simulink model "HT07_accumulator_thermal_model"  (R2022a)
settings: Solver=VariableStepAuto  StartTime=0.0  StopTime=Tend  RelTol=1e-7  AbsTol=1e-7
values from neighbouring files (symbols this model uses):
  AH = 14    [HT07_Simulink_Setup.m]
  SOC0 = 1    [HT07_Simulink_Setup.m]
  startTempC = 25    [HT07_Simulink_Setup.m]
  tabResis = 0.00009    (= 9e-05)    [HT07_Simulink_Setup.m]
undefined symbols (not defined in the file or in its folder): DiscIntNeverNeededParam
libraries: fl_lib x50, nesl_utility x16, ee_lib x2
settings Model: Creator=elrii  LastModifiedBy=David
settings SolverCC: AutoScaleAbsTol=off  AlgebraicLoopSolver=TrustRegion
settings DataIOCC: ReturnWorkspaceOutputsName=tp141c3138_a421_409b_bff7_0e00beb78378
settings DebuggingCC: UnconnectedInputMsg=warning  UnconnectedOutputMsg=warning  UnconnectedLineMsg=warning  SymbolicDimsDataTypeCodeGenerationDiagnostic=none  SFMachineParentedDataDiag=warning
settings SFSimCC: CustomCodeUndefinedFunction=UseInterfaceOnly
settings RTWCC: DLArmComputeVersion=19.05
settings SimscapeCC: SimscapeLogType=all  SimscapeLogSimulationStatistics=on  SimscapeLogDataHistory=10000

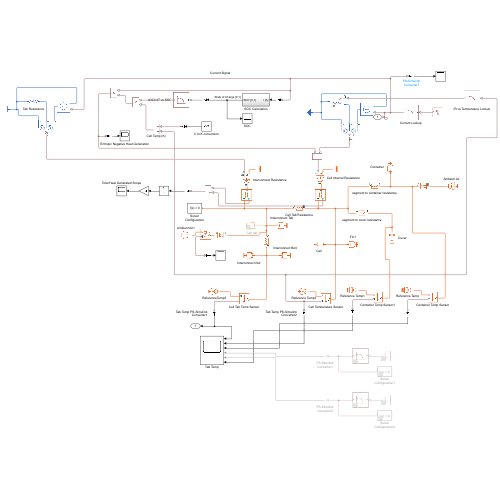
[thumbnail: Simulink's stored preview of the top-level diagram]
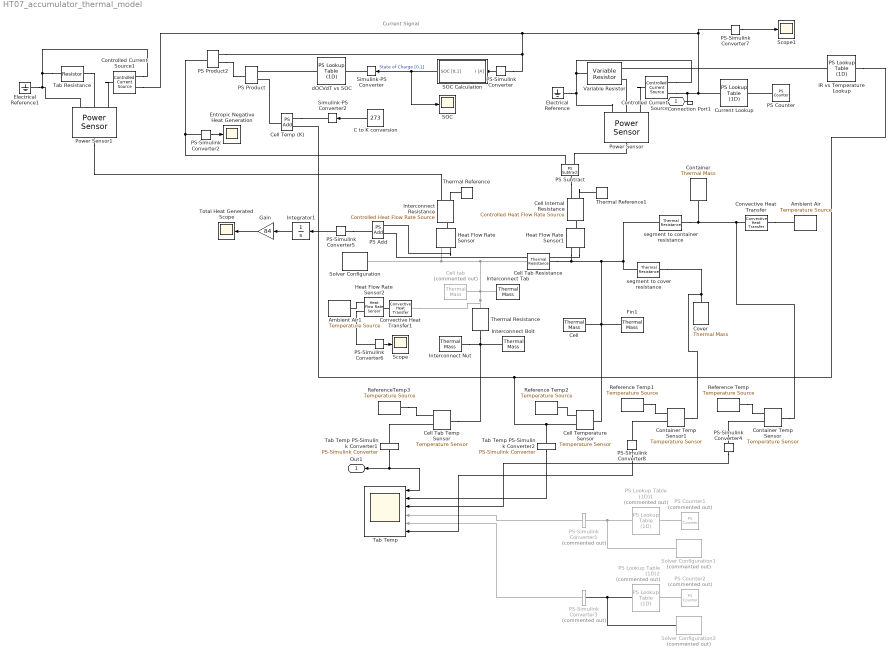
== system HT07_accumulator_thermal_model ==
  note: Current Signal
  " Fin1" : fl_lib/Thermal/Thermal Elements/Thermal Mass  mass=mFin kg  sp_heat=cAl J/kg/K  T_specify=on  T_priority=High  T=startTempC degC  T_nominal_specify=off  T_nominal_unit=K  T_nominal_value=1  Q_specify=off  Q_priority=None  Q=0 W  Q_nominal_specify=off  Q_nominal_unit=W  Q_nominal_value=1
      settings: SourceProductBaseCode=PW,SS,VE
  Ambient Air : fl_lib/Thermal/Thermal Sources/Temperature Source  temperature=startTempC degC
      settings: SourceProductBaseCode=PW,SS,VE
  Ambient Air1 : fl_lib/Thermal/Thermal Sources/Temperature Source  temperature=startTempC degC
      settings: SourceProductBaseCode=PW,SS,VE
  C to K conversion : Constant  Value=273
  "Cell " : fl_lib/Thermal/Thermal Elements/Thermal Mass  mass=mCell kg  sp_heat=cCell J/kg/K  T_specify=on  T_priority=High  T=startTempC degC  T_nominal_specify=off  T_nominal_unit=K  T_nominal_value=1  Q_specify=off  Q_priority=None  Q=0 W  Q_nominal_specify=off  Q_nominal_unit=W  Q_nominal_value=1
      settings: SourceProductBaseCode=PW,SS,VE
  Cell Internal Resistance : fl_lib/Thermal/Thermal Sources/Controlled Heat Flow Rate Source
      settings: SourceProductBaseCode=PW,SS,VE
  Cell Tab Resistance : fl_lib/Thermal/Thermal Elements/Thermal Resistance  resistance=R_tc K/W  T_specify=off  T_priority=None  T=0 K  T_nominal_specify=off  T_nominal_unit=K  T_nominal_value=1  Q_specify=off  Q_priority=None  Q=0 W  Q_nominal_specify=off  Q_nominal_unit=W  Q_nominal_value=1
      settings: SourceProductBaseCode=PW,SS,VE
  Cell Tab Temp Sensor : fl_lib/Thermal/Thermal Sensors/Temperature Sensor
      settings: SourceProductBaseCode=PW,SS,VE
  Cell Temp (K) : fl_lib/Physical Signals/Functions/PS Add
      settings: SourceProductBaseCode=PW,SS,VE
  Cell Temperature Sensor : fl_lib/Thermal/Thermal Sensors/Temperature Sensor
      settings: SourceProductBaseCode=PW,SS,VE
  Cell tab : fl_lib/Thermal/Thermal Elements/Thermal Mass  Commented=on  mass=cellTabThermalMass kg  sp_heat=cCu J/kg/K  T_specify=on  T_priority=High  T=startTempC degC  T_nominal_specify=off  T_nominal_unit=K  T_nominal_value=1  Q_specify=off  Q_priority=None  Q=0 W  Q_nominal_specify=off  Q_nominal_unit=W  Q_nominal_value=1
      settings: SourceProductBaseCode=PW,SS,VE
  Container : fl_lib/Thermal/Thermal Elements/Thermal Mass  mass=mContainerAdj kg  sp_heat=cAl J/kg/K  T_specify=on  T_priority=High  T=startTempC degC  T_nominal_specify=off  T_nominal_unit=K  T_nominal_value=1  Q_specify=off  Q_priority=None  Q=0 W  Q_nominal_specify=off  Q_nominal_unit=W  Q_nominal_value=1
      settings: SourceProductBaseCode=PW,SS,VE
  Container Temp Sensor : fl_lib/Thermal/Thermal Sensors/Temperature Sensor
      settings: SourceProductBaseCode=PW,SS,VE
  Container Temp Sensor1 : fl_lib/Thermal/Thermal Sensors/Temperature Sensor
      settings: SourceProductBaseCode=PW,SS,VE
  Controlled Current Source : fl_lib/Electrical/Electrical Sources/Controlled Current Source
      settings: SourceProductBaseCode=PW,SS,VE
  Controlled Current Source1 : fl_lib/Electrical/Electrical Sources/Controlled Current Source
      settings: SourceProductBaseCode=PW,SS,VE
  Convective Heat Transfer : fl_lib/Thermal/Thermal Elements/Convective Heat Transfer  area=convectionArea m^2  heat_tr_coeff=20 W/(m^2*K)  T_specify=off  T_priority=None  T=0 K  T_nominal_specify=off  T_nominal_unit=K  T_nominal_value=1  Q_specify=off  Q_priority=None  Q=0 W  Q_nominal_specify=off  Q_nominal_unit=W  Q_nominal_value=1
      settings: SourceProductBaseCode=PW,SS,VE
  Convective Heat Transfer1 : fl_lib/Thermal/Thermal Elements/Convective Heat Transfer  area=tabConvectionArea m^2  heat_tr_coeff=100 W/(m^2*K)  T_specify=off  T_priority=None  T=0 K  T_nominal_specify=off  T_nominal_unit=K  T_nominal_value=1  Q_specify=off  Q_priority=None  Q=0 W  Q_nominal_specify=off  Q_nominal_unit=W  Q_nominal_value=1
      settings: SourceProductBaseCode=PW,SS,VE
  Cover : fl_lib/Thermal/Thermal Elements/Thermal Mass  mass=mCoverAdj kg  sp_heat=cAl J/kg/K  T_specify=on  T_priority=High  T=startTempC degC  T_nominal_specify=off  T_nominal_unit=K  T_nominal_value=1  Q_specify=off  Q_priority=None  Q=0 W  Q_nominal_specify=off  Q_nominal_unit=W  Q_nominal_value=1
      settings: SourceProductBaseCode=PW,SS,VE
  Current Lookup : fl_lib/Physical Signals/Lookup Tables/PS Lookup Table (1D)  x=time  f=current A  interp_method=simscape.enum.interpolation.linear  extrap_method=simscape.enum.extrapolation.nearest
      settings: SourceProductBaseCode=PW,SS,VE
  Electrical Reference : fl_lib/Electrical/Electrical Elements/Electrical Reference
      settings: SourceProductBaseCode=PW,SS,VE
  Electrical Reference1 : fl_lib/Electrical/Electrical Elements/Electrical Reference
      settings: SourceProductBaseCode=PW,SS,VE
  Entropic Negative Heat Generation : Scope
  Gain : Gain  Gain=84
  Heat Flow Rate Sensor : fl_lib/Thermal/Thermal Sensors/Heat Flow Rate Sensor
      settings: SourceProductBaseCode=PW,SS,VE
  Heat Flow Rate Sensor1 : fl_lib/Thermal/Thermal Sensors/Heat Flow Rate Sensor
      settings: SourceProductBaseCode=PW,SS,VE
  Heat Flow Rate Sensor2 : fl_lib/Thermal/Thermal Sensors/Heat Flow Rate Sensor
      settings: SourceProductBaseCode=PW,SS,VE
  IR vs Temperature Lookup : fl_lib/Physical Signals/Lookup Tables/PS Lookup Table (1D)  x=tempVec K  f=IRVec Ohm  interp_method=simscape.enum.interpolation.linear  extrap_method=simscape.enum.extrapolation.nearest
      settings: SourceProductBaseCode=PW,SS,VE
  Integrator1 : Integrator
  Interconnect Bolt : fl_lib/Thermal/Thermal Elements/Thermal Mass  mass=mInterconnectBoltTotal kg  sp_heat=cSt J/kg/K  T_specify=on  T_priority=High  T=startTempC degC  T_nominal_specify=off  T_nominal_unit=K  T_nominal_value=1  Q_specify=off  Q_priority=None  Q=0 W  Q_nominal_specify=off  Q_nominal_unit=W  Q_nominal_value=1
      settings: SourceProductBaseCode=PW,SS,VE
  Interconnect Nut : fl_lib/Thermal/Thermal Elements/Thermal Mass  mass=mInterconnectNutTotal kg  sp_heat=cSt J/kg/K  T_specify=on  T_priority=High  T=startTempC degC  T_nominal_specify=off  T_nominal_unit=K  T_nominal_value=1  Q_specify=off  Q_priority=None  Q=0 W  Q_nominal_specify=off  Q_nominal_unit=W  Q_nominal_value=1
      settings: SourceProductBaseCode=PW,SS,VE
  Interconnect Resistance : fl_lib/Thermal/Thermal Sources/Controlled Heat Flow Rate Source
      settings: SourceProductBaseCode=PW,SS,VE
  Interconnect Tab : fl_lib/Thermal/Thermal Elements/Thermal Mass  mass=mInterconnect kg  sp_heat=cAl J/kg/K  T_specify=on  T_priority=High  T=startTempC degC  T_nominal_specify=off  T_nominal_unit=K  T_nominal_value=1  Q_specify=off  Q_priority=None  Q=0 W  Q_nominal_specify=off  Q_nominal_unit=W  Q_nominal_value=1
      settings: SourceProductBaseCode=PW,SS,VE
  PS Add : fl_lib/Physical Signals/Functions/PS Add
      settings: SourceProductBaseCode=PW,SS,VE
  PS Counter : fl_lib/Physical Signals/Sources/PS Counter  sample_time=1 s  init_val=1  reset_val=0  max_val=100000
      settings: SourceProductBaseCode=PW,SS,VE  InternalSimscapePortConfiguration="{\"Bottom\":[],\"Left\":[],\"Right\":[{\"id\":\"Y\",\"label\":\"Y\",\"type\":\"output\"}],\"Top\":[]}"
  PS Counter1 : fl_lib/Physical Signals/Sources/PS Counter  Commented=on  sample_time=1 s  init_val=1  reset_val=0  max_val=100000
      settings: SourceProductBaseCode=PW,SS,VE  InternalSimscapePortConfiguration="{\"Bottom\":[],\"Left\":[],\"Right\":[{\"id\":\"Y\",\"label\":\"Y\",\"type\":\"output\"}],\"Top\":[]}"
  PS Counter2 : fl_lib/Physical Signals/Sources/PS Counter  Commented=on  sample_time=1 s  init_val=1  reset_val=0  max_val=100000
      settings: SourceProductBaseCode=PW,SS,VE  InternalSimscapePortConfiguration="{\"Bottom\":[],\"Left\":[],\"Right\":[{\"id\":\"Y\",\"label\":\"Y\",\"type\":\"output\"}],\"Top\":[]}"
  PS Lookup Table (1D)1 : fl_lib/Physical Signals/Lookup Tables/PS Lookup Table (1D)  Commented=on  x=time  f=tempInterp  interp_method=simscape.enum.interpolation.linear  extrap_method=simscape.enum.extrapolation.nearest
      settings: SourceProductBaseCode=PW,SS,VE
  PS Lookup Table (1D)2 : fl_lib/Physical Signals/Lookup Tables/PS Lookup Table (1D)  Commented=on  x=time  f=accAirTempInterp  interp_method=simscape.enum.interpolation.linear  extrap_method=simscape.enum.extrapolation.nearest
      settings: SourceProductBaseCode=PW,SS,VE
  PS Product : fl_lib/Physical Signals/Functions/PS Product
      settings: SourceProductBaseCode=PW,SS,VE
  PS Product2 : fl_lib/Physical Signals/Functions/PS Product
      settings: SourceProductBaseCode=PW,SS,VE
  PS Subtract : fl_lib/Physical Signals/Functions/PS Subtract
      settings: SourceProductBaseCode=PW,SS,VE
  PS-Simulink Converter{,2,4..5,8} (5 alike) : nesl_utility/PS-Simulink Converter  PhysicalDomain=network_engine_domain  SubClassName=ps_output  LeftPortType=input  RightPortType=output  PseudoPeriodic=off  Frequencies=[]  VectorFormat=1-D array  Unit=inherit  AffineConversion=off
      settings: SourceProductBaseCode=SS,PW,VE
  PS-Simulink Converter1 : nesl_utility/PS-Simulink Converter  Commented=on  PhysicalDomain=network_engine_domain  SubClassName=ps_output  LeftPortType=input  RightPortType=output  PseudoPeriodic=off  Frequencies=[]  VectorFormat=1-D array  Unit=inherit  AffineConversion=off
      settings: SourceProductBaseCode=SS,PW,VE
  PS-Simulink Converter3 : nesl_utility/PS-Simulink Converter  Commented=on  PhysicalDomain=network_engine_domain  SubClassName=ps_output  LeftPortType=input  RightPortType=output  PseudoPeriodic=off  Frequencies=[]  VectorFormat=1-D array  Unit=inherit  AffineConversion=off
      settings: SourceProductBaseCode=SS,PW,VE
  PS-Simulink Converter6 : nesl_utility/PS-Simulink Converter  PhysicalDomain=network_engine_domain  SubClassName=ps_output  LeftPortType=input  RightPortType=output  PseudoPeriodic=off  Frequencies=[]  VectorFormat=inherit  Unit=inherit  AffineConversion=off
      settings: SourceProductBaseCode=SS,PW,VE
  PS-Simulink Converter7 : nesl_utility/PS-Simulink Converter  PhysicalDomain=network_engine_domain  SubClassName=ps_output  LeftPortType=input  RightPortType=output  PseudoPeriodic=off  Frequencies=[]  VectorFormat=inherit  Unit=inherit  AffineConversion=off
      settings: SourceProductBaseCode=SS,PW,VE
  Power Sensor : ee_lib/Sensors & Transducers/Power Sensor  measurement_type=1  averaging_period=1e-4 s
      settings: SourceProductBaseCode=PS
  Power Sensor1 : ee_lib/Sensors & Transducers/Power Sensor  measurement_type=1  averaging_period=1e-4 s
      settings: SourceProductBaseCode=PS
  Reference Temp : fl_lib/Thermal/Thermal Sources/Temperature Source  temperature=0 degC
      settings: SourceProductBaseCode=PW,SS,VE
  Reference Temp1 : fl_lib/Thermal/Thermal Sources/Temperature Source  temperature=0 degC
      settings: SourceProductBaseCode=PW,SS,VE
  Reference Temp2 : fl_lib/Thermal/Thermal Sources/Temperature Source  temperature=0 degC
      settings: SourceProductBaseCode=PW,SS,VE
  ReferenceTemp3 : fl_lib/Thermal/Thermal Sources/Temperature Source  temperature=0 degC
      settings: SourceProductBaseCode=PW,SS,VE
  SOC : Scope
  SOC Calculation : Subsystem
  Scope : Scope
  Scope1 : Scope
  Simulink-PS Converter : nesl_utility/Simulink-PS Converter  PhysicalDomain=network_engine_domain  SubClassName=ps_input  LeftPortType=input  RightPortType=output  PseudoPeriodic=off  Frequencies=[]  NoiseDistribution=none  NoiseParameters=[]  Unit=1  AffineConversion=off  FilteringAndDerivatives=provide  SimscapeFilterOrder=1  InputFilterTimeConstant=0.001  UdotUserProvided=0
      settings: SourceProductBaseCode=SS,PW,VE
  Simulink-PS Converter2 : nesl_utility/Simulink-PS Converter  PhysicalDomain=network_engine_domain  SubClassName=ps_input  LeftPortType=input  RightPortType=output  PseudoPeriodic=off  Frequencies=[]  NoiseDistribution=none  NoiseParameters=[]  Unit=K  AffineConversion=off  FilteringAndDerivatives=provide  SimscapeFilterOrder=1  InputFilterTimeConstant=0.001  UdotUserProvided=0
      settings: SourceProductBaseCode=SS,PW,VE
  Solver Configuration : nesl_utility/Solver Configuration  PhysicalDomain=network_engine_domain  SubClassName=solver  LeftPortType=input  RightPortType=generic  Tones=[]  Harmonics=[]  SimulateNoise=off  Profile=off  UseLocalSampling=off  EnableSwitchedLinearOptims=on  FrequencyDomain=off  UseCCode=off  RelTol=0.001  AbsTol=1e-06  MinStep=1e-09  ToWorkspace=off  RevertToSquareIcSolve=off  NumHomotopyIterations=100  PhasorMode=off  PhasorModeNumHarmonics=1  IndexReductionMethod=DerivativeReplacement  DoDC=off  ResidualTolerance=1e-012  UseLocalSolver=off  LocalSolverChoice=NE_BACKWARD_EULER_ADVANCER  LocalSolverSampleTime=0.001  DoFixedCost=off  MaxNonlinIter=3  MaxModeIter=2  ComputeImpulses=off  ImpulseIterations=2  LinearAlgebra=auto  LinearAlgebraNumThread=0  EquationFormulation=NE_TIME_EF  DelaysMemoryBudget=1024  AutomaticFiltering=on  FilteringTimeConstant=0.001  PartitionStorageMethod=AS_NEEDED  PartitionMemoryBudget=1024  PartitionMethod=ROBUST
      settings: SourceProductBaseCode=SS,PW,VE
  Solver Configuration1 : nesl_utility/Solver Configuration  Commented=on  PhysicalDomain=network_engine_domain  SubClassName=solver  LeftPortType=input  RightPortType=generic  Tones=[]  Harmonics=[]  SimulateNoise=off  Profile=off  UseLocalSampling=off  EnableSwitchedLinearOptims=on  FrequencyDomain=off  UseCCode=off  RelTol=0.001  AbsTol=1e-06  MinStep=1e-09  ToWorkspace=off  RevertToSquareIcSolve=off  NumHomotopyIterations=100  PhasorMode=off  PhasorModeNumHarmonics=1  IndexReductionMethod=DerivativeReplacement  DoDC=off  ResidualTolerance=1e-09  UseLocalSolver=off  LocalSolverChoice=NE_BACKWARD_EULER_ADVANCER  LocalSolverSampleTime=0.001  DoFixedCost=off  MaxNonlinIter=3  MaxModeIter=2  ComputeImpulses=off  ImpulseIterations=2  LinearAlgebra=auto  LinearAlgebraNumThread=0  EquationFormulation=NE_TIME_EF  DelaysMemoryBudget=1024  AutomaticFiltering=on  FilteringTimeConstant=0.001  PartitionStorageMethod=AS_NEEDED  PartitionMemoryBudget=1024  PartitionMethod=ROBUST
      settings: SourceProductBaseCode=SS,PW,VE
  Solver Configuration2 : nesl_utility/Solver Configuration  Commented=on  PhysicalDomain=network_engine_domain  SubClassName=solver  LeftPortType=input  RightPortType=generic  Tones=[]  Harmonics=[]  SimulateNoise=off  Profile=off  UseLocalSampling=off  EnableSwitchedLinearOptims=on  FrequencyDomain=off  UseCCode=off  RelTol=0.001  AbsTol=1e-06  MinStep=1e-09  ToWorkspace=off  RevertToSquareIcSolve=off  NumHomotopyIterations=100  PhasorMode=off  PhasorModeNumHarmonics=1  IndexReductionMethod=DerivativeReplacement  DoDC=off  ResidualTolerance=1e-09  UseLocalSolver=off  LocalSolverChoice=NE_BACKWARD_EULER_ADVANCER  LocalSolverSampleTime=0.001  DoFixedCost=off  MaxNonlinIter=3  MaxModeIter=2  ComputeImpulses=off  ImpulseIterations=2  LinearAlgebra=auto  LinearAlgebraNumThread=0  EquationFormulation=NE_TIME_EF  DelaysMemoryBudget=1024  AutomaticFiltering=on  FilteringTimeConstant=0.001  PartitionStorageMethod=AS_NEEDED  PartitionMemoryBudget=1024  PartitionMethod=ROBUST
      settings: SourceProductBaseCode=SS,PW,VE
  Tab Resistance : fl_lib/Electrical/Electrical Elements/Resistor  R=tabResis Ohm  i_specify=off  i_priority=None  i=0 A  i_nominal_specify=off  i_nominal_unit=A  i_nominal_value=1  v_specify=off  v_priority=None  v=0 V  v_nominal_specify=off  v_nominal_unit=V  v_nominal_value=1  mask(Resistor){}
      settings: SourceProductBaseCode=PW,SS,VE
  Tab Temp : Scope  NumInputPorts=6
  Tab Temp PS-Simulink Converter1 : nesl_utility/PS-Simulink Converter  PhysicalDomain=network_engine_domain  SubClassName=ps_output  LeftPortType=input  RightPortType=output  PseudoPeriodic=off  Frequencies=[]  VectorFormat=1-D array  Unit=inherit  AffineConversion=off
      settings: SourceProductBaseCode=SS,PW,VE
  Tab Temp PS-Simulink Converter2 : nesl_utility/PS-Simulink Converter  PhysicalDomain=network_engine_domain  SubClassName=ps_output  LeftPortType=input  RightPortType=output  PseudoPeriodic=off  Frequencies=[]  VectorFormat=1-D array  Unit=inherit  AffineConversion=off
      settings: SourceProductBaseCode=SS,PW,VE
  Thermal Reference : fl_lib/Thermal/Thermal Elements/Thermal Reference
      settings: SourceProductBaseCode=PW,SS,VE
  Thermal Reference1 : fl_lib/Thermal/Thermal Elements/Thermal Reference
      settings: SourceProductBaseCode=PW,SS,VE
  Thermal Resistance : fl_lib/Thermal/Thermal Elements/Thermal Resistance  resistance=thermistorContactRes K/W  T_specify=off  T_priority=None  T=0 K  T_nominal_specify=off  T_nominal_unit=K  T_nominal_value=1  Q_specify=off  Q_priority=None  Q=0 W  Q_nominal_specify=off  Q_nominal_unit=W  Q_nominal_value=1
      settings: SourceProductBaseCode=PW,SS,VE
  Total Heat Generated Scope : Scope
  Variable Resistor : fl_lib/Electrical/Electrical Elements/Variable Resistor  Rmin=0 Ohm  i_specify=off  i_priority=None  i=0 A  i_nominal_specify=off  i_nominal_unit=A  i_nominal_value=1  v_specify=off  v_priority=None  v=0 V  v_nominal_specify=off  v_nominal_unit=V  v_nominal_value=1
      settings: SourceProductBaseCode=PW,SS,VE
  dOCVdT vs SOC : fl_lib/Physical Signals/Lookup Tables/PS Lookup Table (1D)  x=SOC  f=dOCVdT V/K  interp_method=simscape.enum.interpolation.linear  extrap_method=simscape.enum.extrapolation.nearest
      settings: SourceProductBaseCode=PW,SS,VE
  segment to container resistance : fl_lib/Thermal/Thermal Elements/Thermal Resistance  resistance=R_cb K/W  T_specify=off  T_priority=None  T=0 K  T_nominal_specify=off  T_nominal_unit=K  T_nominal_value=1  Q_specify=off  Q_priority=None  Q=0 W  Q_nominal_specify=off  Q_nominal_unit=W  Q_nominal_value=1
      settings: SourceProductBaseCode=PW,SS,VE
  segment to cover resistance : fl_lib/Thermal/Thermal Elements/Thermal Resistance  resistance=R_cb K/W  T_specify=off  T_priority=None  T=0 K  T_nominal_specify=off  T_nominal_unit=K  T_nominal_value=1  Q_specify=off  Q_priority=None  Q=0 W  Q_nominal_specify=off  Q_nominal_unit=W  Q_nominal_value=1
      settings: SourceProductBaseCode=PW,SS,VE
  Connection Port1 : PMIOPort  Side=Left
  Out1 : Outport
  wires:
  Tab Temp PS-Simulink Converter1/1 -> Tab Temp/1, Out1/1
  PS-Simulink Converter1/1 -> Tab Temp/4
  PS-Simulink Converter/1 -> SOC Calculation/1(I [A])
  SOC Calculation/1(SOC [0,1]) -> Simulink-PS Converter/1, SOC/1  "State of Charge [0,1]"
  C to K conversion/1 -> Simulink-PS Converter2/1
  PS-Simulink Converter2/1 -> Entropic Negative Heat Generation/1
  Tab Temp PS-Simulink Converter2/1 -> Tab Temp/2
  PS-Simulink Converter5/1 -> Integrator1/1
  Integrator1/1 -> Gain/1
  Gain/1 -> Total Heat Generated Scope/1
  PS-Simulink Converter4/1 -> Tab Temp/3
  PS-Simulink Converter3/1 -> Tab Temp/5
  PS-Simulink Converter6/1 -> Scope/1
  PS-Simulink Converter7/1 -> Scope1/1
  PS-Simulink Converter8/1 -> Tab Temp/6
  connections:
  segment to cover resistance/LConn1 -- segment to container resistance/LConn1 -- Heat Flow Rate Sensor1/RConn2 -- Cell Tab Resistance/RConn1 -- Cell Temperature Sensor/LConn1 -- " Fin1"/LConn1 -- "Cell "/LConn1
  Cell tab/LConn1 -- Convective Heat Transfer1/LConn1 -- Thermal Resistance/LConn1 -- Interconnect Tab/LConn1 -- Heat Flow Rate Sensor/RConn2 -- Solver Configuration/RConn1 -- Cell Tab Resistance/LConn1
  Controlled Current Source/LConn1 -- Power Sensor/LConn1
  Power Sensor/LConn2 -- Variable Resistor/LConn2
  Power Sensor/LConn3 -- Electrical Reference/LConn1 -- Controlled Current Source/RConn2 -- Variable Resistor/RConn1
  Tab Resistance/RConn1 -- Controlled Current Source1/RConn2 -- Power Sensor1/LConn3 -- Electrical Reference1/LConn1
  Tab Resistance/LConn1 -- Power Sensor1/LConn2
  Controlled Current Source1/LConn1 -- Power Sensor1/LConn1
  Power Sensor1/RConn1 -- Interconnect Resistance/RConn1
  Interconnect Resistance/RConn2 -- Thermal Reference/LConn1
  segment to container resistance/RConn1 -- Container Temp Sensor/LConn1 -- Convective Heat Transfer/LConn1 -- Container/LConn1
  Controlled Current Source/RConn1 -- Connection Port1/RConn1 -- PS-Simulink Converter7/LConn1 -- PS Product2/LConn1 -- PS-Simulink Converter/LConn1 -- Controlled Current Source1/RConn1 -- Current Lookup/RConn1
  PS Counter/RConn1 -- Current Lookup/LConn1
  ReferenceTemp3/LConn1 -- Cell Tab Temp Sensor/RConn1
  PS Lookup Table (1D)1/RConn1 -- Solver Configuration1/RConn1 -- PS-Simulink Converter1/LConn1
  PS Lookup Table (1D)1/LConn1 -- PS Counter1/RConn1
  Tab Temp PS-Simulink Converter1/LConn1 -- Cell Tab Temp Sensor/RConn2
  Simulink-PS Converter/RConn1 -- dOCVdT vs SOC/LConn1
  dOCVdT vs SOC/RConn1 -- PS Product/LConn1
  PS Product2/LConn2 -- PS Product/RConn1
  PS Subtract/LConn1 -- Power Sensor/RConn1
  PS Subtract/RConn1 -- Cell Internal Resistance/RConn1
  Cell Temp (K)/LConn1 -- Simulink-PS Converter2/RConn1
  Cell Temp (K)/RConn1 -- PS Product/LConn2
  PS-Simulink Converter4/LConn1 -- Container Temp Sensor/RConn2
  Convective Heat Transfer/RConn1 -- Ambient Air/LConn1
  PS Subtract/LConn2 -- PS Product2/RConn1 -- PS-Simulink Converter2/LConn1
  IR vs Temperature Lookup/RConn1 -- Variable Resistor/LConn1
  Cell Temperature Sensor/RConn2 -- Tab Temp PS-Simulink Converter2/LConn1 -- IR vs Temperature Lookup/LConn1 -- Cell Temp (K)/LConn2
  segment to cover resistance/RConn1 -- Container Temp Sensor1/LConn1 -- Cover/LConn1
  Interconnect Nut/LConn1 -- Cell Tab Temp Sensor/LConn1 -- Thermal Resistance/RConn1 -- Interconnect Bolt/LConn1
  Reference Temp/LConn1 -- Container Temp Sensor/RConn1
  Cell Temperature Sensor/RConn1 -- Reference Temp2/LConn1
  Cell Internal Resistance/RConn2 -- Thermal Reference1/LConn1
  Interconnect Resistance/LConn1 -- Heat Flow Rate Sensor/LConn1
  Cell Internal Resistance/LConn1 -- Heat Flow Rate Sensor1/LConn1
  Heat Flow Rate Sensor1/RConn1 -- PS Add/LConn1
  Heat Flow Rate Sensor/RConn1 -- PS Add/LConn2
  PS-Simulink Converter5/LConn1 -- PS Add/RConn1
  PS-Simulink Converter3/LConn1 -- PS Lookup Table (1D)2/RConn1 -- Solver Configuration2/RConn1
  PS Lookup Table (1D)2/LConn1 -- PS Counter2/RConn1
  Convective Heat Transfer1/RConn1 -- Heat Flow Rate Sensor2/LConn1
  Heat Flow Rate Sensor2/RConn2 -- Ambient Air1/LConn1
  Heat Flow Rate Sensor2/RConn1 -- PS-Simulink Converter6/LConn1
  PS-Simulink Converter8/LConn1 -- Container Temp Sensor1/RConn2
  Reference Temp1/LConn1 -- Container Temp Sensor1/RConn1

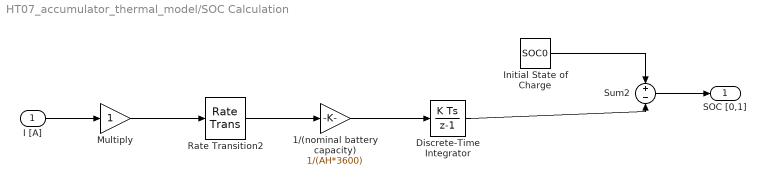
== system HT07_accumulator_thermal_model/SOC Calculation ==
  I [A] : Inport
  1/(nominal battery capacity) : Gain  Gain=1/(AH*3600)
  Discrete-Time Integrator : DiscreteIntegrator  SampleTime=-1  ICPrevOutput=DiscIntNeverNeededParam  ICPrevScaledInput=DiscIntNeverNeededParam
  Initial State of Charge : Constant  Value=SOC0
  Multiply : Gain
  Rate Transition2 : RateTransition
  Sum2 : Sum  Inputs=+-
  SOC [0,1] : Outport  VectorParamsAs1DForOutWhenUnconnected=off
  wires:
  Rate Transition2/1 -> 1/(nominal battery capacity)/1
  1/(nominal battery capacity)/1 -> Discrete-Time Integrator/1
  Initial State of Charge/1 -> Sum2/1
  Discrete-Time Integrator/1 -> Sum2/2
  Sum2/1 -> SOC [0,1]/1
  I [A]/1 -> Multiply/1
  Multiply/1 -> Rate Transition2/1
